simulink model "model_for_report"  (R2013b)
settings: Solver=ode45  StartTime=0.0  StopTime=15  FixedStep=0.01  RelTol=1e-3
values from neighbouring files (symbols this model uses):
  I = 2.1799    [d0.mat]    (also in d1.mat = 1.6541; d2.mat = 1.4039; d3.mat = 1.1608; d4.mat = 1.0272)
  K = 0.0113567305831    [estimation 3b.mat]
  P = 0.42758    [d0.mat]    (also in d1.mat = 0.36594; d2.mat = 0.38394; d3.mat = 0.32408; d4.mat = 0.35291)
  R = 1.0963371881    [estimation 3b.mat]
libraries: fl_lib x9, nesl_utility x4, simulink x1
settings Model: Creator=maen  LastModifiedBy=Nabeel Ahmad
settings SolverCC: AutoInsertRateTranBlk=on
settings DataIOCC: SignalLoggingSaveFormat=ModelDataLogs
settings OptimizationCC: ExpressionDepthLimit=2147483647
settings DebuggingCC: FcnCallInpInsideContextMsg=UseLocalSettings  StateNameClashWarn=warning
settings GRTTargetCC: CombineOutputUpdateFcns=off  GRTInterface=on

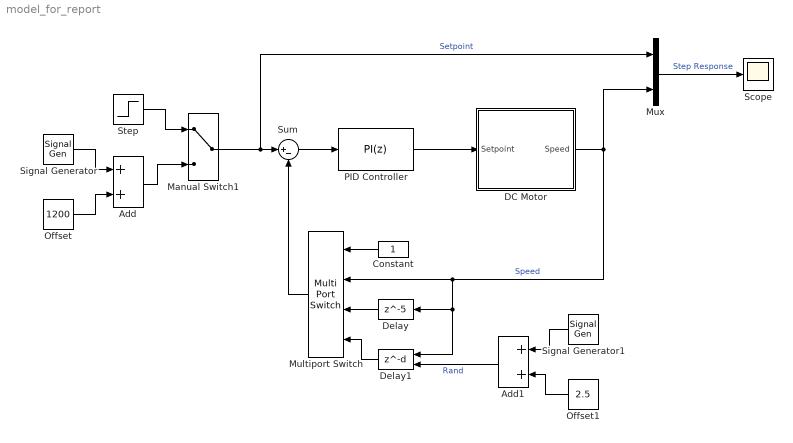
== system model_for_report ==
  Add : Sum
  Add1 : Sum  OutDataTypeStr=uint8
  Constant : Constant
  DC Motor : Subsystem
  Delay : Delay  DelayLength=5  InitialCondition=0  SampleTime=.1
  Delay1 : Delay  DelayLengthSource=Input port  InitialCondition=0  SampleTime=.1
      settings: InputPortMap=u0,p1
  Manual Switch1 : ManualSwitch
  Multiport Switch : MultiPortSwitch
  Mux : Mux  Inputs=2
  Offset : Constant  Value=1200
  Offset1 : Constant  Value=2.5
  PID Controller : simulink/Continuous/PID Controller  Controller=PI  TimeDomain=Discrete-time  SampleTime=.1  IntegratorMethod=Forward Euler  FilterMethod=Forward Euler  Form=Parallel  P=P  I=I  D=-6.78839610676139  N=58.2381885976492  InitialConditionSource=internal  InitialConditionForIntegrator=0  InitialConditionForFilter=0  ExternalReset=none  LimitOutput=on  UpperSaturationLimit=24/K  LowerSaturationLimit=0  LinearizeAsGain=on  AntiWindupMode=none  Kb=1  TrackingMode=off  Kt=1  PParamMin=[]  PParamMax=[]  IParamMin=[]  IParamMax=[]  DParamMin=[]  DParamMax=[]  NParamMin=[]  NParamMax=[]  KbParamMin=[]  KbParamMax=[]  KtParamMin=[]  KtParamMax=[]  POutMin=[]  POutMax=[]  IOutMin=[]  IOutMax=[]  DOutMin=[]  DOutMax=[]  NOutMin=[]  NOutMax=[]  KbOutMin=[]  KbOutMax=[]  KtOutMin=[]  KtOutMax=[]  IntegratorOutMin=[]  IntegratorOutMax=[]  FilterOutMin=[]  FilterOutMax=[]  SumOutMin=[]  SumOutMax=[]  SumI1OutMin=[]  SumI1OutMax=[]  SumI2OutMin=[]  SumI2OutMax=[]  SumI3OutMin=[]  SumI3OutMax=[]  SumDOutMin=[]  SumDOutMax=[]  SaturationOutMin=[]  SaturationOutMax=[]  IntegratorContinuousStateAttributes=''  IntegratorStateMustResolveToSignalObject=off  IntegratorRTWStateStorageClass=Auto  FilterContinuousStateAttributes=''  FilterStateMustResolveToSignalObject=off  FilterRTWStateStorageClass=Auto
  Scope : Scope
      settings: TimeRange=15  YMin=0  YMax=2500
  Signal Generator : SignalGenerator  Amplitude=400  Frequency=.2
  Signal Generator1 : SignalGenerator  Amplitude=2.5  Frequency=.05
  Step : Step  Time=2  After=1500  SampleTime=0
  Sum : Sum  Inputs=|+-
  wires:
  Mux/1 -> Scope/1  "Step Response"
  PID Controller/1 -> DC Motor/1(Setpoint)
  Sum/1 -> PID Controller/1
  Manual Switch1/1 -> Mux/1, Sum/1  "Setpoint"
  Add/1 -> Manual Switch1/2
  Signal Generator/1 -> Add/1
  Offset/1 -> Add/2
  Step/1 -> Manual Switch1/1
  Delay/1 -> Multiport Switch/3
  Constant/1 -> Multiport Switch/1
  Delay1/1 -> Multiport Switch/4
  DC Motor/1(" Speed") -> Delay1/1, Delay/1, Multiport Switch/2, Mux/2  "Speed"
  Multiport Switch/1 -> Sum/2
  Offset1/1 -> Add1/2
  Signal Generator1/1 -> Add1/1
  Add1/1 -> Delay1/2  "Rand"

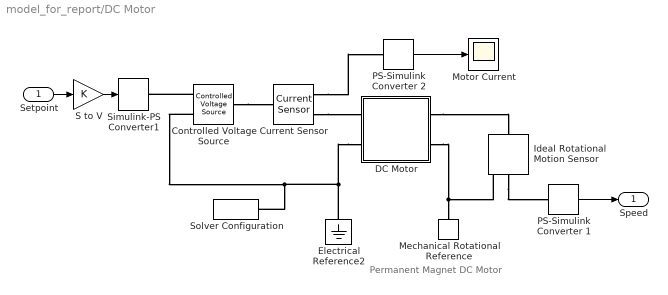
== system model_for_report/DC Motor ==
  note: Permanent Magnet DC Motor
  Setpoint : Inport
  Controlled Voltage Source : fl_lib/Electrical/Electrical Sources/Controlled Voltage Source  i_Log=off  v_Log=off  LocalVarNames=|i|v  LocalVarDescs=|i|v  LocalVarLogging=[0 0]
  Current Sensor : fl_lib/Electrical/Electrical Sensors/Current Sensor  i1_Log=off  v1_Log=off  LocalVarNames=|i1|v1  LocalVarDescs=|i1|v1  LocalVarLogging=[]
  DC Motor : Subsystem
  Electrical Reference2 : fl_lib/Electrical/Electrical Elements/Electrical Reference  i_Log=off  LocalVarNames=|i  LocalVarDescs=|i  LocalVarLogging=[]
  Ideal Rotational Motion Sensor : fl_lib/Mechanical/Mechanical Sensors/Ideal Rotational Motion Sensor  offset=0 rad  w_Log=off  t_Log=off  phi_Log=off  LocalVarNames=|w|t|phi  LocalVarDescs=|w|t|phi  LocalVarLogging=[]
  Mechanical Rotational Reference : fl_lib/Mechanical/Rotational Elements/Mechanical Rotational Reference  t_Log=off  LocalVarNames=|t  LocalVarDescs=|t  LocalVarLogging=[]
  Motor Current : Scope
      settings: YMin=0  YMax=2.25
  PS-Simulink Converter 1 : nesl_utility/PS-Simulink Converter  PhysicalDomain=network_engine_domain  SubClassName=ps_output  LeftPortType=input  RightPortType=output  PseudoPeriodic=off  Frequencies=[]  Unit=rpm  AffineConversion=off
  PS-Simulink Converter 2 : nesl_utility/PS-Simulink Converter  PhysicalDomain=network_engine_domain  SubClassName=ps_output  LeftPortType=input  RightPortType=output  PseudoPeriodic=off  Frequencies=[]  Unit=1  AffineConversion=off
  S to V : Gain  Gain=K
  Simulink-PS Converter1 : nesl_utility/Simulink-PS Converter  PhysicalDomain=network_engine_domain  SubClassName=ps_input  LeftPortType=input  RightPortType=output  PseudoPeriodic=off  Frequencies=[]  NoiseDistribution=none  NoiseParameters=[]  Unit=V  AffineConversion=off  InputFiltering=off  SimscapeFilterOrder=1  InputFilterTimeConstant=.001  UdotUserProvided=0
  Solver Configuration : nesl_utility/Solver Configuration  PhysicalDomain=network_engine_domain  SubClassName=solver  LeftPortType=input  RightPortType=generic  Accelerate=off  Tones=[]  Harmonics=[]  SimulateNoise=off  Profile=off  UseLocalSampling=off  EnableSwitchedLinearOptims=on  FrequencyDomain=off  UseCCode=off  RelTol=0.001  AbsTol=1e-06  MinStep=1e-09  ToWorkspace=off  DoDC=off  ResidualTolerance=1e-9  UseLocalSolver=off  LocalSolverChoice=NE_BACKWARD_EULER_ADVANCER  LocalSolverSampleTime=.001  DoFixedCost=off  MaxNonlinIter=3  MaxModeIter=2  LinearAlgebra=Sparse  DelaysMemoryBudget=1024
  " Speed" : Outport
  wires:
  PS-Simulink Converter 2/1 -> Motor Current/1
  PS-Simulink Converter 1/1 -> " Speed"/1
  Setpoint/1 -> S to V/1
  S to V/1 -> Simulink-PS Converter1/1
  connections:
  DC Motor/LConn2 -- Electrical Reference2/LConn1 -- Controlled Voltage Source/RConn2 -- Solver Configuration/RConn1
  Ideal Rotational Motion Sensor/RConn1 -- DC Motor/RConn2 -- Mechanical Rotational Reference/LConn1
  Current Sensor/RConn2 -- DC Motor/LConn1
  Ideal Rotational Motion Sensor/RConn2 -- PS-Simulink Converter 1/LConn1
  Current Sensor/RConn1 -- PS-Simulink Converter 2/LConn1
  Controlled Voltage Source/LConn1 -- Current Sensor/LConn1
  DC Motor/RConn1 -- Ideal Rotational Motion Sensor/LConn1
  Controlled Voltage Source/RConn1 -- Simulink-PS Converter1/RConn1

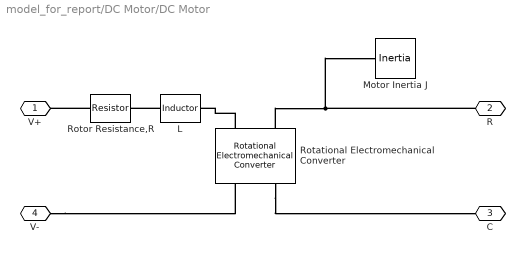
== system model_for_report/DC Motor/DC Motor ==
  L : fl_lib/Electrical/Electrical Elements/Inductor  l=L H  i0=0 A  r=0 Ohm  g=1e-09 1/Ohm  i_Log=off  v_Log=off  i_L_Log=off  LocalVarNames=|current|voltage|power  LocalVarDescs=|Inductor current (A) |Voltage across inductor (V)|Power (W)  LocalVarLogging=[0 0 0]
  Motor Inertia J : fl_lib/Mechanical/Rotational Elements/Inertia  inertia=J kg*m^2  initial_velocity=0 rad/s  t_Log=off  LocalVarNames=|torque|velocity  LocalVarDescs=|Inertia torque (N*m)|Inertia absolute velocity (rad/s)  LocalVarLogging=[0 0]
  Rotational Electromechanical Converter : fl_lib/Electrical/Electrical Elements/Rotational Electromechanical Converter  K=K V/rpm  i_Log=off  v_Log=off  t_Log=off  w_Log=off  LocalVarNames=|current|voltage|power|torque|speed  LocalVarDescs=|Current (A)|Voltage (V)|Power (W)|Torque (Nm)|Angular speed (rad/s)  LocalVarLogging=[0 0 0 0 0]
  Rotor Resistance,R : fl_lib/Electrical/Electrical Elements/Resistor  Tag=Factory Generic  R=R Ohm  i_Log=off  v_Log=off  LocalVarNames=|current|voltage|power  LocalVarDescs=|Resistor current (A)|Voltage across resistor (V)|Power (W)  LocalVarLogging=[0 0 0]
  V+ : PMIOPort  Port=1  Side=Left
  R : PMIOPort  Port=2  Side=Right
  C : PMIOPort  Port=3  Side=Right
  V- : PMIOPort  Port=4  Side=Left
  connections:
  Rotational Electromechanical Converter/LConn1 -- L/RConn1
  V-/RConn1 -- Rotational Electromechanical Converter/RConn1
  Rotor Resistance,R/LConn1 -- V+/RConn1
  L/LConn1 -- Rotor Resistance,R/RConn1
  Rotational Electromechanical Converter/LConn2 -- R/RConn1 -- Motor Inertia J/LConn1
  Rotational Electromechanical Converter/RConn2 -- C/RConn1
